simulink model "Bebop10_from_exp"  (R2018a)
settings: Solver=VariableStepAuto  StartTime=0.0  StopTime=100  FixedStep=0.0025  MaxStep=1  MinStep=0.005  RelTol=10  AbsTol=10
values from neighbouring files (symbols this model uses):
  flightplan = [dist,0,height,deg2rad(090) ... (first row only)    [compare_cubic_spline_1.m]    (also in initialize_race_realtime.m = flightplan - [0.5*min(flightplan(:,1:2))+0.5*max(flightplan(; initialize_race_realtime_backup_cubic.m; plot_sim.m = [ 4.348, -0.278, height, deg2rad(  0); test_b_spline.m)
  FOV = 1.05    [initialize_race_realtime_backup_cubic.m]
  g = 9.81    [initialize_race_no_realtime.m]    (also in initialize_race_realtime.m; initialize_race_realtime_backup_cubic.m; moving_average_rls_own.m = P(i-1)*meas*(lambda+meas*P(i-1)*meas)^-1)
  gate_size = 1.4    [initialize_race_realtime.m]    (also in initialize_race_realtime_backup_cubic.m)
  gates = sim_gates(:,:,1)    [eval_sim.m]    (also in initialize_race_realtime.m = flightplan + pert; initialize_race_realtime_backup_cubic.m = [dist,0,height,deg2rad(110); plot_sim.m)
  HFOV = VFOV*resolution(1)/resolution(2)    [initialize_race_realtime.m]
  I = [1 0 0 ... (first row only)    [Bebop_sim_init.m]    (also in initialize_race_no_realtime.m; initialize_race_realtime.m; initialize_race_realtime_backup_cubic.m; moving_averge_rls_download.m = ones(1,N))
  m = 0.68    [calc_plot_spline.m]    (also in calc_spline.m; compare_cubic_spline_1.m = vpasolve(e,r); compare_cubic_spline_2.m = r/3*(-sin(dp)+sqrt(sin(dp)^2-6*cos(dp)+6)); initialize_race_no_realtime.m = 2)
  mass = 2    [Bebop_sim_init.m]    (also in initialize_race_realtime.m = 0.5)
  max_rot_Z = (90)*pi/180    (= 1.57079632679)    [Bebop_sim_init.m]    (also in initialize_race_no_realtime.m = 1.0471975512; initialize_race_realtime.m = 3.14159265359; initialize_race_realtime_backup_cubic.m; run_batch1.m = list_agility(idx_agility)*max_rot_Z)
  max_theta_X = (40)*pi/180    (= 0.698131700798)    [Bebop_sim_init.m]    (also in initialize_race_no_realtime.m = 0.13962634016; initialize_race_realtime.m = 0.418879020479; initialize_race_realtime_backup_cubic.m = 1.308996939; run_batch1.m = list_agility(idx_agility)*max_theta_X)
  max_theta_Y = (40)*pi/180    (= 0.698131700798)    [Bebop_sim_init.m]    (also in initialize_race_no_realtime.m = 0.13962634016; initialize_race_realtime.m = 0.418879020479; initialize_race_realtime_backup_cubic.m = 1.308996939; run_batch1.m = list_agility(idx_agility)*max_theta_Y)
  max_v_Z = .5    (= 0.5)    [Bebop_sim_init.m]    (also in initialize_race_no_realtime.m = 1; initialize_race_realtime.m = 6; initialize_race_realtime_backup_cubic.m = 3; run_batch1.m = list_agility(idx_agility)*max_v_Z)
  max_vel = 2.0    (= 2)    [initialize_race_realtime.m]    (also in initialize_race_realtime_backup_cubic.m = 1.5; run_batch1.m = list_speed(idx_speed); run_batch2.m = list_speed(idx_speed); run_batch3.m = list_speed(idx_speed))
  resolution = 0.5*[1280 720]    [initialize_race_realtime.m]
  spline_init = [P0;P1;P2;P3]    [initialize_race_realtime.m]
  std_dev_eul = 0.25*deg2rad(0.8)*ones(1,3)    [initialize_race_realtime.m]    (also in run_batch1.m = list_sensor_eul(idx_sensor)*dist*ones(1,3); run_batch2.m = list_sensor_eul(idx_sensor)*dist*ones(1,3); run_batch3.m = list_sensor_eul(idx_sensor)*dist*ones(1,3); run_batch4.m = list_sensor_eul(idx_sensor)*dist*ones(1,3))
  std_dev_F = 0.1*max_force*ones(1,3)    [initialize_race_realtime.m]    (also in run_batch1.m = list_actuator(idx_actuator)*max_force*ones(1,3); run_batch2.m = list_actuator(idx_actuator)*max_force*ones(1,3); run_batch3.m = list_actuator(idx_sensor)*max_force*ones(1,3); run_batch4.m = list_actuator(idx_sensor)*max_force*ones(1,3))
  std_dev_M = 0.1*max_moment*[0, 0, 1]    [initialize_race_realtime.m]    (also in run_batch1.m = list_actuator(idx_actuator)*max_moment*[0, 0, 1]; run_batch2.m = list_actuator(idx_actuator)*max_moment*[0, 0, 1]; run_batch3.m = list_actuator(idx_sensor)*max_moment*[0, 0, 1]; run_batch4.m = list_actuator(idx_sensor)*max_moment*[0, 0, 1])
  std_dev_vel = 0.06*ones(1,3)    [initialize_race_realtime.m]    (also in run_batch1.m = list_sensor(idx_sensor)*dist*ones(1,3); run_batch2.m = list_sensor(idx_sensor)*dist*ones(1,3); run_batch3.m = list_sensor(idx_sensor)*dist*ones(1,3); run_batch4.m = list_sensor(idx_sensor)*dist*ones(1,3))
  std_dev_xyz = 0.06*ones(1,3)    [initialize_race_realtime.m]    (also in run_batch1.m = list_sensor(idx_sensor)*dist*ones(1,3); run_batch2.m = list_sensor(idx_sensor)*dist*ones(1,3); run_batch3.m = list_sensor(idx_sensor)*dist*ones(1,3); run_batch4.m = list_sensor(idx_sensor)*dist*ones(1,3))
  two_std_dev_init = [1,1,0.5,deg2rad(30)]    [initialize_race_realtime.m]
  two_std_dev_thres = 0.3    [initialize_race_realtime.m]
  VFOV = 1.05    [initialize_race_realtime.m]
undefined symbols (not defined in the file or in its folder): gray, Rec, SDTV
libraries: sharedtransform x13, visiontextngfix x5, aerolibactuator x4, simulink x3, aerolibutil x2, visionconversions x2, shared6dof x1, vrlib x1, visionanalysis x1, visionstatistics x1, visiontransforms x1
(part 2 of 3)

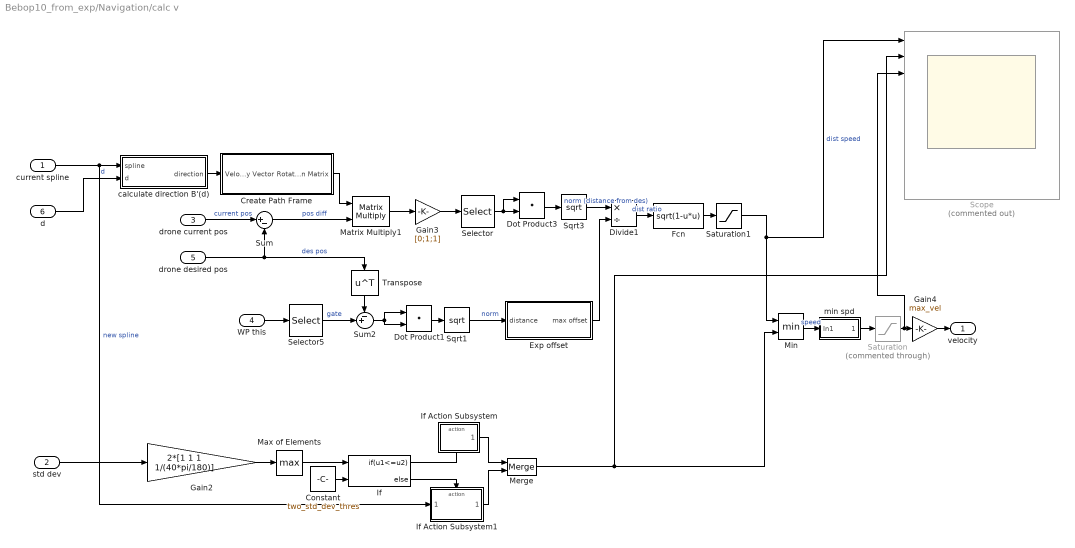
== system Bebop10_from_exp/Navigation/calc v ==
  current spline : Inport
  std dev : Inport  Port=2
  drone current pos : Inport  Port=3
  WP this : Inport  Port=4
  drone desired pos : Inport  Port=5
  d : Inport  Port=6
  Constant : Constant  Value=two_std_dev_thres
  Create Path Frame : Subsystem
  Divide1 : Product  Inputs=*/
  Dot Product1 : DotProduct  InputSameDT=on  OutDataTypeStr=Inherit: Inherit via internal rule
  Dot Product3 : DotProduct  InputSameDT=on  OutDataTypeStr=Inherit: Inherit via internal rule
  Exp offset : Subsystem
  Fcn : Fcn  Expr=sqrt(1-u*u)
  Gain2 : Gain  Gain=2*[1 1 1 1/(40*pi/180)]
  Gain3 : Gain  Gain=[0;1;1]
  Gain4 : Gain  Gain=max_vel
  If : If  NumInputs=2  IfExpression=u1<=u2
  If Action Subsystem : Subsystem  TreatAsAtomicUnit=on
  If Action Subsystem1 : Subsystem  TreatAsAtomicUnit=on
  Matrix Multiply1 : Product  Inputs=**  Multiplication=Matrix(*)
  Max of Elements : MinMax  Function=max
  Merge : Merge
  Min : MinMax  Inputs=2
  Saturation : Saturate  Commented=through  UpperLimit=1.01  LowerLimit=0.99
  Saturation1 : Saturate  UpperLimit=1  LowerLimit=0
  Scope : Scope  Commented=on  NumInputPorts=10
  Selector : Selector  IndexMode=Zero-based  InputPortWidth=3  IndexOptions=Index vector (dialog)  Indices=[0 1 2]  OutputSizes=1
  Selector5 : Selector  NumberOfDimensions=2  IndexMode=Zero-based  InputPortWidth=4  IndexOptions=Select all,Index vector (dialog)  Indices=[1 2 3],[0 1 2]  OutputSizes=1,1
  Sqrt1 : Sqrt  SaturateOnIntegerOverflow=on
  Sqrt3 : Sqrt  SaturateOnIntegerOverflow=on
  Sum : Sum  Inputs=|+-
  Sum2 : Sum  Inputs=-+|
  Transpose : Math  Operator=transpose  SaturateOnIntegerOverflow=on
  calculate direction B'(d) : Subsystem
  min spd : Subsystem
  velocity : Outport
  wires:
  If Action Subsystem1/1(red vel) -> Merge/2
  If Action Subsystem/1(1) -> Merge/1
  If/1 -> If Action Subsystem/Action
  std dev/1 -> Gain2/1
  If/2 -> If Action Subsystem1/Action
  Gain2/1 -> Max of Elements/1
  Max of Elements/1 -> If/1
  Create Path Frame/1(Rotation Matrix) -> Matrix Multiply1/1
  Sum2/1 -> Dot Product1/1, Dot Product1/2
  Min/1 -> min spd/1(In1)  "speed"
  Fcn/1 -> Saturation1/1
  Saturation/1 -> Scope/3, Gain4/1
  Dot Product3/1 -> Sqrt3/1
  Selector5/1 -> Sum2/2  "gate"
  calculate direction B'(d)/1(direction) -> Create Path Frame/1(Velocity Vector)
  Divide1/1 -> Fcn/1  "dist ratio"
  Selector/1 -> Dot Product3/1, Dot Product3/2
  d/1 -> calculate direction B'(d)/2(d)  "d"
  Sum/1 -> Matrix Multiply1/2  "pos diff"
  Merge/1 -> Scope/2, Min/2
  Sqrt1/1 -> Exp offset/1(distance)  "norm"
  Dot Product1/1 -> Sqrt1/1
  drone desired pos/1 -> Transpose/1, Sum/2  "des pos"
  Saturation1/1 -> Scope/1, Min/1  "dist speed"
  Exp offset/1(max offset) -> Divide1/2
  Gain4/1 -> velocity/1
  Sqrt3/1 -> Divide1/1  "norm (distance from des)"
  drone current pos/1 -> Sum/1  "current pos"
  Transpose/1 -> Sum2/1
  min spd/1(Out1) -> Saturation/1
  Matrix Multiply1/1 -> Gain3/1
  current spline/1 -> If Action Subsystem1/1(spline), calculate direction B'(d)/1(spline)  "new spline"
  WP this/1 -> Selector5/1
  Constant/1 -> If/2
  Gain3/1 -> Selector/1

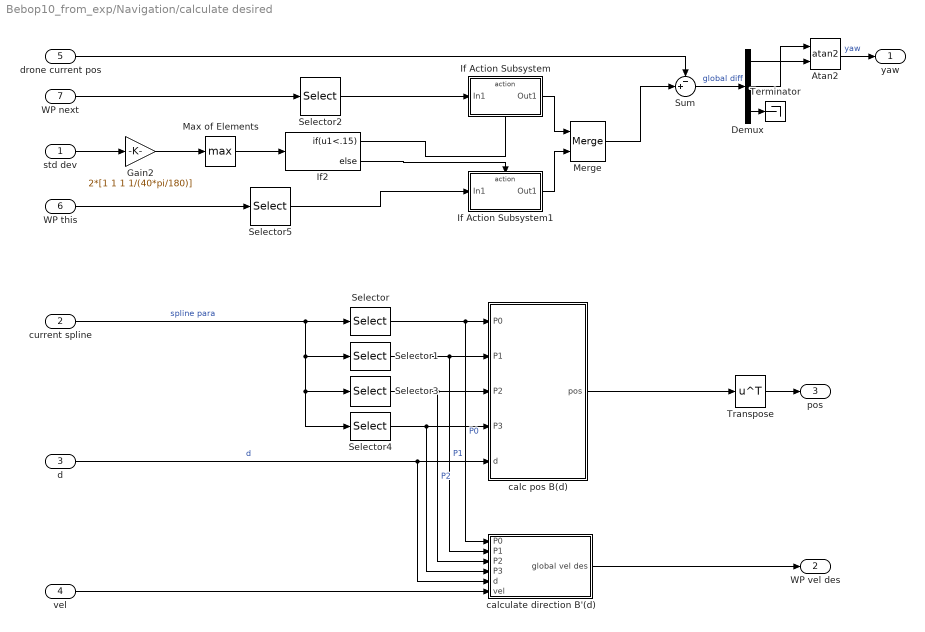
== system Bebop10_from_exp/Navigation/calculate desired ==
  std dev : Inport
  current spline : Inport  Port=2
  d : Inport  Port=3
  vel : Inport  Port=4
  drone current pos : Inport  Port=5
  WP this : Inport  Port=6
  WP next : Inport  Port=7
  Atan2 : Trigonometry  Operator=atan2
  Demux : Demux  Outputs=3
  Gain2 : Gain  Gain=2*[1 1 1 1/(40*pi/180)]
  If Action Subsystem : Subsystem  TreatAsAtomicUnit=on
  If Action Subsystem1 : Subsystem  TreatAsAtomicUnit=on
  If2 : If  IfExpression=u1<.15
  Max of Elements : MinMax  Function=max
  Merge : Merge
  Selector : Selector  NumberOfDimensions=2  IndexMode=Zero-based  InputPortWidth=3  IndexOptions=Index vector (dialog),Select all  Indices=0,[0 1 2]  OutputSizes=1,1
  Selector1 : Selector  NumberOfDimensions=2  IndexMode=Zero-based  InputPortWidth=3  IndexOptions=Index vector (dialog),Select all  Indices=1,[0 1 2]  OutputSizes=1,1
  Selector2 : Selector  NumberOfDimensions=2  IndexMode=Zero-based  InputPortWidth=4  IndexOptions=Select all,Index vector (dialog)  Indices=[1 2 3],[0 1 2]  OutputSizes=1,1
  Selector3 : Selector  NumberOfDimensions=2  IndexMode=Zero-based  InputPortWidth=3  IndexOptions=Index vector (dialog),Select all  Indices=2,[0 1 2]  OutputSizes=1,1
  Selector4 : Selector  NumberOfDimensions=2  IndexMode=Zero-based  InputPortWidth=3  IndexOptions=Index vector (dialog),Select all  Indices=3,[0 1 2]  OutputSizes=1,1
  Selector5 : Selector  NumberOfDimensions=2  IndexMode=Zero-based  InputPortWidth=4  IndexOptions=Select all,Index vector (dialog)  Indices=[1 2 3],[0 1 2]  OutputSizes=1,1
  Sum : Sum  Inputs=-+|
  Terminator : Terminator
  Transpose : Math  Operator=transpose  SaturateOnIntegerOverflow=on
  calc pos B(d) : Subsystem
  calculate direction B'(d) : Subsystem
  yaw : Outport
  WP vel des : Outport  Port=2
  pos : Outport  Port=3
  wires:
  current spline/1 -> Selector4/1, Selector3/1, Selector1/1, Selector/1  "spline para"
  Selector/1 -> calculate direction B'(d)/1(P0), calc pos B(d)/1(P0)  "P0"
  Selector1/1 -> calculate direction B'(d)/2(P1), calc pos B(d)/2(P1)  "P1"
  Selector3/1 -> calculate direction B'(d)/3(P2), calc pos B(d)/3(P2)  "P2"
  d/1 -> calc pos B(d)/5(d), calculate direction B'(d)/5(d)  "d"
  calc pos B(d)/1(pos) -> Transpose/1
  Sum/1 -> Demux/1  "global diff"
  Demux/2 -> Atan2/1
  Demux/1 -> Atan2/2
  Demux/3 -> Terminator/1
  Atan2/1 -> yaw/1  "yaw"
  vel/1 -> calculate direction B'(d)/6(vel)
  calculate direction B'(d)/1(global vel des) -> WP vel des/1
  Transpose/1 -> pos/1
  drone current pos/1 -> Sum/1
  WP next/1 -> Selector2/1
  If Action Subsystem/1(Out1) -> Merge/1
  If Action Subsystem1/1(Out1) -> Merge/2
  WP this/1 -> Selector5/1
  Selector2/1 -> If Action Subsystem/1(In1)
  Selector4/1 -> calc pos B(d)/4(P3), calculate direction B'(d)/4(P3)
  Merge/1 -> Sum/2
  std dev/1 -> Gain2/1
  Gain2/1 -> Max of Elements/1
  Max of Elements/1 -> If2/1
  If2/1 -> If Action Subsystem/Action
  Selector5/1 -> If Action Subsystem1/1(In1)
  If2/2 -> If Action Subsystem1/Action

== system Bebop10_from_exp/Navigation/get WPts ==
  list : Inport
  idx : Inport  Port=2
  Fcn : Fcn  Expr=u-1
  Fcn1 : Fcn  Expr=u+1
  Mod : Math  Operator=mod  SaturateOnIntegerOverflow=on
  Mod1 : Math  Operator=mod  SaturateOnIntegerOverflow=on
  Mod2 : Math  Operator=mod  SaturateOnIntegerOverflow=on
  Probe Dimension : Probe  ProbeWidth=off  ProbeSampleTime=off  ProbeComplexSignal=off  ProbeSignalDimensions=on
  Selector : Selector  InputPortWidth=2  IndexOptions=Index vector (dialog)  Indices=1  OutputSizes=1
  Selector1 : Selector  NumberOfDimensions=2  IndexMode=Zero-based  InputPortWidth=3  IndexOptions=Index vector (port),Select all  Indices=[1 3],1  OutputSizes=1,1
  Selector2 : Selector  NumberOfDimensions=2  IndexMode=Zero-based  InputPortWidth=3  IndexOptions=Index vector (port),Select all  Indices=[1 3],1  OutputSizes=1,1
  Selector3 : Selector  NumberOfDimensions=2  IndexMode=Zero-based  InputPortWidth=3  IndexOptions=Index vector (port),Select all  Indices=[1 3],1  OutputSizes=1,1
  WP last : Outport
  WP this : Outport  Port=2
  WP next : Outport  Port=3
  wires:
  list/1 -> Selector3/1, Selector2/1, Selector1/1, Probe Dimension/1
  idx/1 -> Fcn/1, Mod1/1, Fcn1/1
  Fcn/1 -> Mod/1
  Mod/1 -> Selector1/2
  Fcn1/1 -> Mod2/1
  Probe Dimension/1 -> Selector/1
  Selector/1 -> Mod2/2, Mod1/2, Mod/2
  Mod1/1 -> Selector2/2
  Mod2/1 -> Selector3/2
  Selector1/1 -> WP last/1
  Selector2/1 -> WP this/1
  Selector3/1 -> WP next/1

== system Bebop10_from_exp/Navigation/set position ==
  current spline : Inport
  velocity : Inport  Port=2
  d old : Inport  Port=3
  auto : Inport  Port=4
  Constant2 : Constant
  Mod1 : Math  Operator=mod  SaturateOnIntegerOverflow=on
  Selector10 : Selector  NumberOfDimensions=2  IndexMode=Zero-based  InputPortWidth=3  IndexOptions=Index vector (dialog),Select all  Indices=1,[0 1 2]  OutputSizes=1,1
  Selector11 : Selector  NumberOfDimensions=2  IndexMode=Zero-based  InputPortWidth=3  IndexOptions=Index vector (dialog),Select all  Indices=2,[0 1 2]  OutputSizes=1,1
  Selector12 : Selector  NumberOfDimensions=2  IndexMode=Zero-based  InputPortWidth=3  IndexOptions=Index vector (dialog),Select all  Indices=3,[0 1 2]  OutputSizes=1,1
  Selector7 : Selector  NumberOfDimensions=2  IndexMode=Zero-based  InputPortWidth=3  IndexOptions=Index vector (dialog),Select all  Indices=0,[0 1 2]  OutputSizes=1,1
  Unit Delay2 : UnitDelay  SampleTime=-1
  new d with linearization : Subsystem
  d old1 : Outport
  d new raw : Outport  Port=2
  wires:
  current spline/1 -> Selector7/1, Selector10/1, Selector11/1, Selector12/1  "spline para"
  Selector7/1 -> new d with linearization/3(P0)  "P0"
  Selector10/1 -> new d with linearization/4(P1)  "P1"
  Selector11/1 -> new d with linearization/5(P2)  "P2"
  Selector12/1 -> new d with linearization/6(P3)  "P3"
  d old/1 -> new d with linearization/2(d old)
  velocity/1 -> new d with linearization/1(vel)
  new d with linearization/1(d new same spline) -> d new raw/1, Mod1/1  "d new over"
  Mod1/1 -> Unit Delay2/1
  Constant2/1 -> Mod1/2
  Unit Delay2/1 -> d old1/1
  auto/1 -> new d with linearization/7(auto)

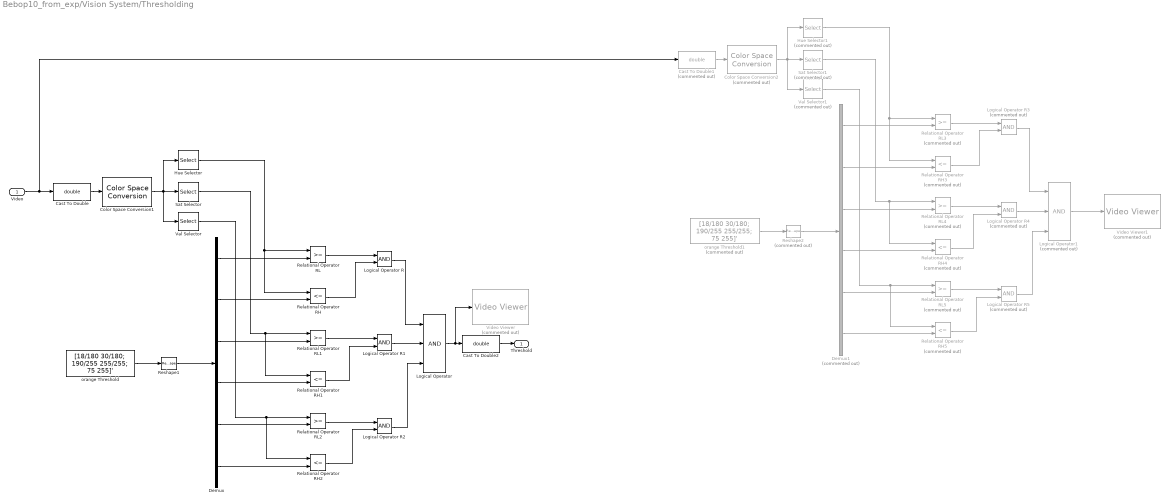
== system Bebop10_from_exp/Vision System/Thresholding ==
  "Video " : Inport
  Cast To Double : DataTypeConversion  OutDataTypeStr=double
  Cast To Double1 : DataTypeConversion  Commented=on  OutDataTypeStr=double
  Cast To Double2 : DataTypeConversion  OutDataTypeStr=double
  Color Space Conversion1 : visionconversions/Color Space  Conversion  conversion=Obsolete  conversionActive=R'G'B' to HSV  wp_str=D65  rec=Rec. 601 (SDTV)  sys=1125/60/2:1  imagePorts=One multidimensional signal
      settings: SourceProductName=Computer Vision System Toolbox
  Color Space Conversion2 : visionconversions/Color Space  Conversion  Commented=on  conversion=Obsolete  conversionActive=R'G'B' to HSV  wp_str=D65  rec=Rec. 601 (SDTV)  sys=1125/60/2:1  imagePorts=One multidimensional signal
      settings: SourceProductName=Computer Vision System Toolbox
  Demux : Demux  Outputs=6
  Demux1 : Demux  Commented=on  Outputs=6
  Hue Selector : Selector  NumberOfDimensions=3  IndexMode=Zero-based  InputPortWidth=3  IndexOptions=Select all,Select all,Index vector (dialog)  Indices=[1 3],1,0  OutputSizes=1,1,1
  Hue Selector1 : Selector  Commented=on  NumberOfDimensions=3  InputPortWidth=3  IndexOptions=Select all,Select all,Index vector (dialog)  Indices=[1 3],1,1  OutputSizes=1,1,1
  Logical Operator : Logic  Inputs=3  AllPortsSameDT=off  OutDataTypeStr=boolean
  Logical Operator R : Logic  AllPortsSameDT=off  OutDataTypeStr=boolean
  Logical Operator R1 : Logic  AllPortsSameDT=off  OutDataTypeStr=boolean
  Logical Operator R2 : Logic  AllPortsSameDT=off  OutDataTypeStr=boolean
  Logical Operator R3 : Logic  Commented=on  AllPortsSameDT=off  OutDataTypeStr=boolean
  Logical Operator R4 : Logic  Commented=on  AllPortsSameDT=off  OutDataTypeStr=boolean
  Logical Operator R5 : Logic  Commented=on  AllPortsSameDT=off  OutDataTypeStr=boolean
  Logical Operator1 : Logic  Commented=on  Inputs=3  AllPortsSameDT=off  OutDataTypeStr=boolean
  Relational Operator RH : RelationalOperator  Operator=<=  OutDataTypeStr=boolean  RndMeth=Nearest
  Relational Operator RH1 : RelationalOperator  Operator=<=  OutDataTypeStr=boolean  RndMeth=Nearest
  Relational Operator RH2 : RelationalOperator  Operator=<=  OutDataTypeStr=boolean  RndMeth=Nearest
  Relational Operator RH3 : RelationalOperator  Commented=on  Operator=<=  OutDataTypeStr=boolean  RndMeth=Nearest
  Relational Operator RH4 : RelationalOperator  Commented=on  Operator=<=  OutDataTypeStr=boolean  RndMeth=Nearest
  Relational Operator RH5 : RelationalOperator  Commented=on  Operator=<=  OutDataTypeStr=boolean  RndMeth=Nearest
  Relational Operator RL : RelationalOperator  OutDataTypeStr=boolean  RndMeth=Nearest
  Relational Operator RL1 : RelationalOperator  OutDataTypeStr=boolean  RndMeth=Nearest
  Relational Operator RL2 : RelationalOperator  OutDataTypeStr=boolean  RndMeth=Nearest
  Relational Operator RL3 : RelationalOperator  Commented=on  OutDataTypeStr=boolean  RndMeth=Nearest
  Relational Operator RL4 : RelationalOperator  Commented=on  OutDataTypeStr=boolean  RndMeth=Nearest
  Relational Operator RL5 : RelationalOperator  Commented=on  OutDataTypeStr=boolean  RndMeth=Nearest
  Reshape1 : Reshape
  Reshape2 : Reshape  Commented=on
  Sat Selector : Selector  NumberOfDimensions=3  IndexMode=Zero-based  InputPortWidth=3  IndexOptions=Select all,Select all,Index vector (dialog)  Indices=[1 3],1,1  OutputSizes=1,1,1
  Sat Selector1 : Selector  Commented=on  NumberOfDimensions=3  InputPortWidth=3  IndexOptions=Select all,Select all,Index vector (dialog)  Indices=[1 3],1,2  OutputSizes=1,1,1
  Val Selector : Selector  NumberOfDimensions=3  IndexMode=Zero-based  InputPortWidth=3  IndexOptions=Select all,Select all,Index vector (dialog)  Indices=[1 3],1,2  OutputSizes=1,1,1
  Val Selector1 : Selector  Commented=on  NumberOfDimensions=3  InputPortWidth=3  IndexOptions=Select all,Select all,Index vector (dialog)  Indices=[1 3],1,3  OutputSizes=1,1,1
  Video Viewer : VideoViewer  Commented=on  colormapValue=gray(256)  FigPos=[833 898 768 793]
  Video Viewer1 : VideoViewer  Commented=on  colormapValue=gray(256)  FigPos=[823 898 778 793]
  orange Threshold : Constant  Value=[18/180 30/180; 190/255 255/255; 75 255]'  OutDataTypeStr=double
  orange Threshold1 : Constant  Commented=on  Value=[18/180 30/180; 190/255 255/255; 75 255]'  OutDataTypeStr=double
  Threshold : Outport
  wires:
  Color Space Conversion1/1 -> Val Selector/1, Sat Selector/1, Hue Selector/1
  Demux/6 -> Relational Operator RH2/2
  Val Selector/1 -> Relational Operator RH2/1, Relational Operator RL2/1
  Demux/3 -> Relational Operator RL1/2
  Relational Operator RL/1 -> Logical Operator R/1
  Demux/2 -> Relational Operator RH/2
  orange Threshold/1 -> Reshape1/1
  Cast To Double/1 -> Color Space Conversion1/1
  Demux/5 -> Relational Operator RL2/2
  Hue Selector/1 -> Relational Operator RH/1, Relational Operator RL/1
  Logical Operator R/1 -> Logical Operator/1
  Relational Operator RH/1 -> Logical Operator R/2
  Demux/1 -> Relational Operator RL/2
  Demux/4 -> Relational Operator RH1/2
  Reshape1/1 -> Demux/1
  Logical Operator R1/1 -> Logical Operator/2
  Relational Operator RH1/1 -> Logical Operator R1/2
  Sat Selector/1 -> Relational Operator RH1/1, Relational Operator RL1/1
  Relational Operator RL1/1 -> Logical Operator R1/1
  Relational Operator RH2/1 -> Logical Operator R2/2
  Relational Operator RL2/1 -> Logical Operator R2/1
  Logical Operator R2/1 -> Logical Operator/3
  Logical Operator/1 -> Video Viewer/1, Cast To Double2/1
  Demux1/5 -> Relational Operator RL5/2
  Relational Operator RH3/1 -> Logical Operator R3/2
  orange Threshold1/1 -> Reshape2/1
  Demux1/1 -> Relational Operator RL3/2
  Relational Operator RH4/1 -> Logical Operator R4/2
  Demux1/4 -> Relational Operator RH4/2
  Relational Operator RH5/1 -> Logical Operator R5/2
  Logical Operator R5/1 -> Logical Operator1/3
  Relational Operator RL4/1 -> Logical Operator R4/1
  Demux1/6 -> Relational Operator RH5/2
  Demux1/2 -> Relational Operator RH3/2
  Reshape2/1 -> Demux1/1
  Logical Operator1/1 -> Video Viewer1/1
  Hue Selector1/1 -> Relational Operator RH3/1, Relational Operator RL3/1
  Color Space Conversion2/1 -> Val Selector1/1, Sat Selector1/1, Hue Selector1/1
  Logical Operator R3/1 -> Logical Operator1/1
  Cast To Double1/1 -> Color Space Conversion2/1
  Demux1/3 -> Relational Operator RL4/2
  Relational Operator RL3/1 -> Logical Operator R3/1
  Val Selector1/1 -> Relational Operator RH5/1, Relational Operator RL5/1
  Relational Operator RL5/1 -> Logical Operator R5/1
  Logical Operator R4/1 -> Logical Operator1/2
  "Video "/1 -> Cast To Double1/1, Cast To Double/1
  Sat Selector1/1 -> Relational Operator RH4/1, Relational Operator RL4/1
  Cast To Double2/1 -> Threshold/1

== system Bebop10_from_exp/Vision System/show all lines ==
  original image : Inport
  lines : Inport  Port=2
  pts : Inport  Port=3
  Cast To Double : DataTypeConversion  OutDataTypeStr=int32
  Cast To Double1 : DataTypeConversion  OutDataTypeStr=int32
  Draw Markers2 : visiontextngfix/Draw Markers  shape=Circle  size=3  fill=on  fillClrSource=Specify via dialog  display=Black  intensity=200  color=[200 255 100]  opacity=1  viewport=Entire image  antialiasing=off  inType=Obsolete  imagePorts=One multidimensional signal  prodOutputMode=Binary point scaling  prodOutputWordLength=32  prodOutputFracLength=14  memoryMode=Specify word length  memoryWordLength=16  memoryFracLength=14  roundingMode=Floor  overflowMode=off
      settings: SourceProductName=Computer Vision System Toolbox  SourceProductBaseCode=VP
  Draw Shapes : visiontextngfix/Draw Shapes  shape=Lines  fill=off  lineWidth=1  fillClrSource=Specify via dialog  display=White  intensity=200  color=[200 255 100]  opacity=0.6  viewport=Entire image  antialiasing=off  inType=Obsolete  imagePorts=One multidimensional signal  prodOutputMode=Binary point scaling  prodOutputWordLength=32  prodOutputFracLength=14  memoryMode=Specify word length  memoryWordLength=16  memoryFracLength=14  roundingMode=Floor  overflowMode=off
      settings: SourceProductName=Computer Vision System Toolbox
  Video Viewer3 : VideoViewer  colormapValue=gray(256)  FigPos=[66 1078 1855 973]
  wires:
  original image/1 -> Draw Shapes/1
  Draw Shapes/1 -> Draw Markers2/1
  lines/1 -> Cast To Double/1
  pts/1 -> Cast To Double1/1
  Cast To Double/1 -> Draw Shapes/2
  Draw Markers2/1 -> Video Viewer3/1
  Cast To Double1/1 -> Draw Markers2/2

== system Bebop10_from_exp/Vision System/show feature lines ==
  original image : Inport
  lines : Inport  Port=2
  pts : Inport  Port=3
  Cast To Double : DataTypeConversion  OutDataTypeStr=int32
  Cast To Double1 : DataTypeConversion  OutDataTypeStr=int32
  Draw Markers2 : visiontextngfix/Draw Markers  shape=Circle  size=3  fill=on  fillClrSource=Specify via dialog  display=Black  intensity=200  color=[200 255 100]  opacity=1  viewport=Entire image  antialiasing=off  inType=Obsolete  imagePorts=One multidimensional signal  prodOutputMode=Binary point scaling  prodOutputWordLength=32  prodOutputFracLength=14  memoryMode=Specify word length  memoryWordLength=16  memoryFracLength=14  roundingMode=Floor  overflowMode=off
      settings: SourceProductName=Computer Vision System Toolbox  SourceProductBaseCode=VP
  Draw Shapes : visiontextngfix/Draw Shapes  shape=Lines  fill=off  lineWidth=1  fillClrSource=Specify via dialog  display=White  intensity=200  color=[200 255 100]  opacity=0.6  viewport=Entire image  antialiasing=off  inType=Obsolete  imagePorts=One multidimensional signal  prodOutputMode=Binary point scaling  prodOutputWordLength=32  prodOutputFracLength=14  memoryMode=Specify word length  memoryWordLength=16  memoryFracLength=14  roundingMode=Floor  overflowMode=off
      settings: SourceProductName=Computer Vision System Toolbox
  Video Viewer3 : VideoViewer  colormapValue=gray(256)  FigPos=[66 1078 928 945]
  wires:
  original image/1 -> Draw Shapes/1
  Draw Shapes/1 -> Draw Markers2/1
  lines/1 -> Cast To Double/1
  pts/1 -> Cast To Double1/1
  Cast To Double/1 -> Draw Shapes/2
  Draw Markers2/1 -> Video Viewer3/1
  Cast To Double1/1 -> Draw Markers2/2

== system Bebop10_from_exp/Vision System/show gate ==
  original image : Inport
  gate pts : Inport  Port=2
  Draw Markers1 : visiontextngfix/Draw Markers  shape=Circle  size=10  fill=on  fillClrSource=Specify via dialog  display=White  intensity=200  color=[200 255 100]  opacity=1  viewport=Entire image  antialiasing=off  inType=Obsolete  imagePorts=One multidimensional signal  prodOutputMode=Binary point scaling  prodOutputWordLength=32  prodOutputFracLength=14  memoryMode=Specify word length  memoryWordLength=16  memoryFracLength=14  roundingMode=Floor  overflowMode=off
      settings: SourceProductName=Computer Vision System Toolbox  SourceProductBaseCode=VP
  Video Viewer1 : VideoViewer  colormapValue=gray(256)  FigPos=[1104 1072 735 551]
  wires:
  gate pts/1 -> Draw Markers1/2
  Draw Markers1/1 -> Video Viewer1/1
  original image/1 -> Draw Markers1/1

== system Bebop10_from_exp/conv/global2strange drone ==
  note: rotm2axang(m1*m2)
  note: eul2rotm([-pi/2, 0, pi/2])
  note: eul2rotm([euler(3),euler(2),euler(1)])
  euler global : Inport
  Constant : Constant  Value=pi/2
  Constant1 : Constant  Value=0
  Direction Cosine Matrix to Quaternions : sharedtransform/Direction Cosine Matrix  to Quaternions  aMode=0  action=None  tolerance=eps(2)
      settings: SourceProductName=Aerospace Blockset  SourceProductBaseCode=AE
  Gain : Gain  Gain=-1
  Gain2 : Gain  Gain=-1
  Gain3 : Gain  Gain=[-1,-1,-1,1]
  MATLAB Function : MATLAB Function  Commented=on  TreatAsAtomicUnit=on
  MATLAB Function1 : MATLAB Function  TreatAsAtomicUnit=on
  Matrix Multiply : Product  Multiplication=Matrix(*)
  Rotation Angles to Direction Cosine Matrix : sharedtransform/Rotation Angles to Direction Cosine Matrix  rotationOrder=XYZ  aMode=aMode
      settings: SourceProductBaseCode=AE
  Rotation Angles to Direction Cosine Matrix1 : sharedtransform/Rotation Angles to Direction Cosine Matrix  rotationOrder=XYZ  aMode=aMode
      settings: SourceProductBaseCode=AE
  Vector Concatenate : Concatenate  NumInputs=3
  axang strange : Outport
  wires:
  Constant/1 -> Vector Concatenate/3, Gain/1
  Constant1/1 -> Vector Concatenate/2
  Gain/1 -> Vector Concatenate/1
  Rotation Angles to Direction Cosine Matrix/1 -> Matrix Multiply/2
  euler global/1 -> Gain2/1
  Rotation Angles to Direction Cosine Matrix1/1 -> Matrix Multiply/1
  Matrix Multiply/1 -> Direction Cosine Matrix to Quaternions/1
  MATLAB Function1/1(axang) -> Gain3/1
  Vector Concatenate/1 -> Rotation Angles to Direction Cosine Matrix/1
  Gain2/1 -> Rotation Angles to Direction Cosine Matrix1/1
  Direction Cosine Matrix to Quaternions/1 -> MATLAB Function1/1(q)
  Gain3/1 -> axang strange/1

== system Bebop10_from_exp/Control/Create Path Frame/Make X Vector ==
  Velocity Vector : Inport
  Make Unit : Subsystem
  X Vector : Outport
  wires:
  Velocity Vector/1 -> Make Unit/1(Vector)
  Make Unit/1(Unit Vector) -> X Vector/1

== system Bebop10_from_exp/Control/Create Path Frame/Make Y Vector ==
  Velocity Vector : Inport
  Constant : Constant  Value=0
  Demux : Demux  Outputs=3
  Gain : Gain  Gain=-1
  Make Unit : Subsystem
  Matrix Concatenate : Concatenate  NumInputs=3  Mode=Multidimensional array
  Terminator : Terminator
  Y Vector : Outport
  wires:
  Make Unit/1(Unit Vector) -> Y Vector/1
  Velocity Vector/1 -> Demux/1
  Demux/3 -> Terminator/1
  Demux/2 -> Gain/1
  Gain/1 -> Matrix Concatenate/1
  Demux/1 -> Matrix Concatenate/2
  Constant/1 -> Matrix Concatenate/3
  Matrix Concatenate/1 -> Make Unit/1(Vector)

== system Bebop10_from_exp/Control/Create Path Frame/Make Z Vector ==
  Velocity Vector : Inport
  Add : Sum
  Demux : Demux  Outputs=3
  Gain : Gain  Gain=-1
  Gain1 : Gain  Gain=-1
  Make Unit : Subsystem
  Matrix Concatenate : Concatenate  NumInputs=3  Mode=Multidimensional array
  Multiply : Product
  Multiply1 : Product
  Square : Math  Operator=square  SaturateOnIntegerOverflow=on
  Square1 : Math  Operator=square  SaturateOnIntegerOverflow=on
  Z Vector : Outport
  wires:
  Make Unit/1(Unit Vector) -> Z Vector/1
  Velocity Vector/1 -> Demux/1
  Demux/3 -> Multiply/2, Multiply1/2
  Matrix Concatenate/1 -> Make Unit/1(Vector)
  Multiply/1 -> Gain/1
  Gain/1 -> Matrix Concatenate/1
  Demux/1 -> Square/1, Multiply/1
  Multiply1/1 -> Gain1/1
  Gain1/1 -> Matrix Concatenate/2
  Demux/2 -> Square1/1, Multiply1/1
  Add/1 -> Matrix Concatenate/3
  Square/1 -> Add/1
  Square1/1 -> Add/2

== system Bebop10_from_exp/Control/Subsystem/ctrl r ==
  P : Inport
  D : Inport  Port=2
  Value : Inport  Port=3
  Add : Sum  Inputs=+++
  Add1 : Sum
  Gain : Gain  Gain=3
  Gain1 : Gain
  Gain2 : Gain  Gain=2
  Gain3 : Gain  Gain=0.1
  Multiply : Product
  Multiply1 : Product
  Sum : Sum  Inputs=-+|
  Sum1 : Sum  Inputs=-+|
  Sum2 : Sum  Inputs=-+|
  Unit Delay1 : UnitDelay  SampleTime=-1
  Unit Delay2 : UnitDelay  SampleTime=-1
  Unit Delay3 : UnitDelay  SampleTime=-1
  Acc : Outport
  wires:
  Unit Delay1/1 -> Sum/1, Unit Delay2/1
  Multiply1/1 -> Add1/2  "P"
  Multiply/1 -> Sum/2, Sum1/2, Sum2/2, Unit Delay1/1
  Gain3/1 -> Add1/1  "D"
  Unit Delay2/1 -> Sum1/1, Unit Delay3/1
  Value/1 -> Multiply1/1, Multiply/2
  Unit Delay3/1 -> Sum2/1
  Add1/1 -> Acc/1
  D/1 -> Multiply/1
  P/1 -> Multiply1/2
  Sum2/1 -> Gain1/1
  Sum1/1 -> Gain2/1
  Sum/1 -> Gain/1
  Gain1/1 -> Add/1
  Gain2/1 -> Add/2
  Gain/1 -> Add/3
  Add/1 -> Gain3/1

== system Bebop10_from_exp/Control/Subsystem/ctrl x ==
  P : Inport
  D : Inport  Port=2
  Value : Inport  Port=3
  Add : Sum  Inputs=+++
  Add1 : Sum
  Gain : Gain  Gain=3
  Gain1 : Gain
  Gain2 : Gain  Gain=2
  Gain3 : Gain  Gain=0.1
  Multiply : Product
  Multiply1 : Product
  Scope : Scope  NumInputPorts=2
  Sum : Sum  Inputs=-+|
  Sum1 : Sum  Inputs=-+|
  Sum2 : Sum  Inputs=-+|
  Unit Delay1 : UnitDelay  SampleTime=-1
  Unit Delay2 : UnitDelay  SampleTime=-1
  Unit Delay3 : UnitDelay  SampleTime=-1
  Acc : Outport
  wires:
  Unit Delay1/1 -> Sum/1, Unit Delay2/1
  Multiply1/1 -> Scope/2, Add1/2  "P"
  Multiply/1 -> Sum/2, Sum1/2, Sum2/2, Unit Delay1/1
  Gain3/1 -> Scope/1, Add1/1  "D"
  Unit Delay2/1 -> Sum1/1, Unit Delay3/1
  Value/1 -> Multiply1/1, Multiply/2
  Unit Delay3/1 -> Sum2/1
  Add1/1 -> Acc/1
  D/1 -> Multiply/1
  P/1 -> Multiply1/2
  Sum2/1 -> Gain1/1
  Sum1/1 -> Gain2/1
  Sum/1 -> Gain/1
  Gain1/1 -> Add/1
  Gain2/1 -> Add/2
  Gain/1 -> Add/3
  Add/1 -> Gain3/1

== system Bebop10_from_exp/Control/Subsystem/ctrl y ==
  P : Inport
  D : Inport  Port=2
  Value : Inport  Port=3
  Add : Sum  Inputs=+++
  Add1 : Sum
  Gain : Gain  Gain=3
  Gain1 : Gain
  Gain2 : Gain  Gain=2
  Gain3 : Gain  Gain=0.1
  Multiply : Product
  Multiply1 : Product
  Sum : Sum  Inputs=-+|
  Sum1 : Sum  Inputs=-+|
  Sum2 : Sum  Inputs=-+|
  Unit Delay1 : UnitDelay  SampleTime=-1
  Unit Delay2 : UnitDelay  SampleTime=-1
  Unit Delay3 : UnitDelay  SampleTime=-1
  Acc : Outport
  wires:
  Unit Delay1/1 -> Sum/1, Unit Delay2/1
  Multiply1/1 -> Add1/2  "P"
  Multiply/1 -> Sum/2, Sum1/2, Sum2/2, Unit Delay1/1
  Gain3/1 -> Add1/1  "D"
  Unit Delay2/1 -> Sum1/1, Unit Delay3/1
  Value/1 -> Multiply1/1, Multiply/2
  Unit Delay3/1 -> Sum2/1
  Add1/1 -> Acc/1
  D/1 -> Multiply/1
  P/1 -> Multiply1/2
  Sum2/1 -> Gain1/1
  Sum1/1 -> Gain2/1
  Sum/1 -> Gain/1
  Gain1/1 -> Add/1
  Gain2/1 -> Add/2
  Gain/1 -> Add/3
  Add/1 -> Gain3/1

== system Bebop10_from_exp/Control/Subsystem/ctrl z ==
  P : Inport
  D : Inport  Port=2
  Value : Inport  Port=3
  Add : Sum  Inputs=+++
  Add1 : Sum
  Gain : Gain  Gain=3
  Gain1 : Gain
  Gain2 : Gain  Gain=2
  Gain3 : Gain  Gain=0.1
  Multiply : Product
  Multiply1 : Product
  Sum : Sum  Inputs=-+|
  Sum1 : Sum  Inputs=-+|
  Sum2 : Sum  Inputs=-+|
  Unit Delay1 : UnitDelay  SampleTime=-1
  Unit Delay2 : UnitDelay  SampleTime=-1
  Unit Delay3 : UnitDelay  SampleTime=-1
  Acc : Outport
  wires:
  Unit Delay1/1 -> Sum/1, Unit Delay2/1
  Multiply1/1 -> Add1/2  "P"
  Multiply/1 -> Sum/2, Sum1/2, Sum2/2, Unit Delay1/1
  Gain3/1 -> Add1/1  "D"
  Unit Delay2/1 -> Sum1/1, Unit Delay3/1
  Value/1 -> Multiply1/1, Multiply/2
  Unit Delay3/1 -> Sum2/1
  Add1/1 -> Acc/1
  D/1 -> Multiply/1
  P/1 -> Multiply1/2
  Sum2/1 -> Gain1/1
  Sum1/1 -> Gain2/1
  Sum/1 -> Gain/1
  Gain1/1 -> Add/1
  Gain2/1 -> Add/2
  Gain/1 -> Add/3
  Add/1 -> Gain3/1

== system Bebop10_from_exp/Gate info/Yaw2Axang1/Subsystem ==
  note: u(2)/sqrt(1-u(1)*u(1)), u(3)/sqrt(1-u(1)*u(1)), u(4)/sqrt(1-u(1)*u(1)),
  In1 : Inport
  Fcn : Fcn  Expr=2*acos(u(1))
  Fcn1 : Fcn  Expr=u(2)/sqrt(1-u(1)*u(1))
  Fcn2 : Fcn  Expr=u(3)/sqrt(1-u(1)*u(1))
  Fcn3 : Fcn  Expr=u(4)/sqrt(1-u(1)*u(1))
  Vector Concatenate : Concatenate  NumInputs=4
  Out1 : Outport
  wires:
  In1/1 -> Fcn/1, Fcn3/1, Fcn2/1, Fcn1/1
  Fcn1/1 -> Vector Concatenate/1
  Fcn2/1 -> Vector Concatenate/2
  Fcn3/1 -> Vector Concatenate/3
  Fcn/1 -> Vector Concatenate/4
  Vector Concatenate/1 -> Out1/1

== system Bebop10_from_exp/Gate info/Yaw2Axang2/Subsystem ==
  note: u(2)/sqrt(1-u(1)*u(1)), u(3)/sqrt(1-u(1)*u(1)), u(4)/sqrt(1-u(1)*u(1)),
  In1 : Inport
  Fcn : Fcn  Expr=2*acos(u(1))
  Fcn1 : Fcn  Expr=u(2)/sqrt(1-u(1)*u(1))
  Fcn2 : Fcn  Expr=u(3)/sqrt(1-u(1)*u(1))
  Fcn3 : Fcn  Expr=u(4)/sqrt(1-u(1)*u(1))
  Vector Concatenate : Concatenate  NumInputs=4
  Out1 : Outport
  wires:
  In1/1 -> Fcn/1, Fcn3/1, Fcn2/1, Fcn1/1
  Fcn1/1 -> Vector Concatenate/1
  Fcn2/1 -> Vector Concatenate/2
  Fcn3/1 -> Vector Concatenate/3
  Fcn/1 -> Vector Concatenate/4
  Vector Concatenate/1 -> Out1/1

== system Bebop10_from_exp/Gate info/Yaw2Axang3/Subsystem ==
  note: u(2)/sqrt(1-u(1)*u(1)), u(3)/sqrt(1-u(1)*u(1)), u(4)/sqrt(1-u(1)*u(1)),
  In1 : Inport
  Fcn : Fcn  Expr=2*acos(u(1))
  Fcn1 : Fcn  Expr=u(2)/sqrt(1-u(1)*u(1))
  Fcn2 : Fcn  Expr=u(3)/sqrt(1-u(1)*u(1))
  Fcn3 : Fcn  Expr=u(4)/sqrt(1-u(1)*u(1))
  Vector Concatenate : Concatenate  NumInputs=4
  Out1 : Outport
  wires:
  In1/1 -> Fcn/1, Fcn3/1, Fcn2/1, Fcn1/1
  Fcn1/1 -> Vector Concatenate/1
  Fcn2/1 -> Vector Concatenate/2
  Fcn3/1 -> Vector Concatenate/3
  Fcn/1 -> Vector Concatenate/4
  Vector Concatenate/1 -> Out1/1

== system Bebop10_from_exp/Gate info/Yaw2Axang4/Subsystem ==
  note: u(2)/sqrt(1-u(1)*u(1)), u(3)/sqrt(1-u(1)*u(1)), u(4)/sqrt(1-u(1)*u(1)),
  In1 : Inport
  Fcn : Fcn  Expr=2*acos(u(1))
  Fcn1 : Fcn  Expr=u(2)/sqrt(1-u(1)*u(1))
  Fcn2 : Fcn  Expr=u(3)/sqrt(1-u(1)*u(1))
  Fcn3 : Fcn  Expr=u(4)/sqrt(1-u(1)*u(1))
  Vector Concatenate : Concatenate  NumInputs=4
  Out1 : Outport
  wires:
  In1/1 -> Fcn/1, Fcn3/1, Fcn2/1, Fcn1/1
  Fcn1/1 -> Vector Concatenate/1
  Fcn2/1 -> Vector Concatenate/2
  Fcn3/1 -> Vector Concatenate/3
  Fcn/1 -> Vector Concatenate/4
  Vector Concatenate/1 -> Out1/1

== system Bebop10_from_exp/Gate info/Yaw2Axang5/Subsystem ==
  note: u(2)/sqrt(1-u(1)*u(1)), u(3)/sqrt(1-u(1)*u(1)), u(4)/sqrt(1-u(1)*u(1)),
  In1 : Inport
  Fcn : Fcn  Expr=2*acos(u(1))
  Fcn1 : Fcn  Expr=u(2)/sqrt(1-u(1)*u(1))
  Fcn2 : Fcn  Expr=u(3)/sqrt(1-u(1)*u(1))
  Fcn3 : Fcn  Expr=u(4)/sqrt(1-u(1)*u(1))
  Vector Concatenate : Concatenate  NumInputs=4
  Out1 : Outport
  wires:
  In1/1 -> Fcn/1, Fcn3/1, Fcn2/1, Fcn1/1
  Fcn1/1 -> Vector Concatenate/1
  Fcn2/1 -> Vector Concatenate/2
  Fcn3/1 -> Vector Concatenate/3
  Fcn/1 -> Vector Concatenate/4
  Vector Concatenate/1 -> Out1/1

== system Bebop10_from_exp/Gate info/Yaw2Axang6/Subsystem ==
  note: u(2)/sqrt(1-u(1)*u(1)), u(3)/sqrt(1-u(1)*u(1)), u(4)/sqrt(1-u(1)*u(1)),
  In1 : Inport
  Fcn : Fcn  Expr=2*acos(u(1))
  Fcn1 : Fcn  Expr=u(2)/sqrt(1-u(1)*u(1))
  Fcn2 : Fcn  Expr=u(3)/sqrt(1-u(1)*u(1))
  Fcn3 : Fcn  Expr=u(4)/sqrt(1-u(1)*u(1))
  Vector Concatenate : Concatenate  NumInputs=4
  Out1 : Outport
  wires:
  In1/1 -> Fcn/1, Fcn3/1, Fcn2/1, Fcn1/1
  Fcn1/1 -> Vector Concatenate/1
  Fcn2/1 -> Vector Concatenate/2
  Fcn3/1 -> Vector Concatenate/3
  Fcn/1 -> Vector Concatenate/4
  Vector Concatenate/1 -> Out1/1

== system Bebop10_from_exp/Gate info/Yaw2Axang7/Subsystem ==
  note: u(2)/sqrt(1-u(1)*u(1)), u(3)/sqrt(1-u(1)*u(1)), u(4)/sqrt(1-u(1)*u(1)),
  In1 : Inport
  Fcn : Fcn  Expr=2*acos(u(1))
  Fcn1 : Fcn  Expr=u(2)/sqrt(1-u(1)*u(1))
  Fcn2 : Fcn  Expr=u(3)/sqrt(1-u(1)*u(1))
  Fcn3 : Fcn  Expr=u(4)/sqrt(1-u(1)*u(1))
  Vector Concatenate : Concatenate  NumInputs=4
  Out1 : Outport
  wires:
  In1/1 -> Fcn/1, Fcn3/1, Fcn2/1, Fcn1/1
  Fcn1/1 -> Vector Concatenate/1
  Fcn2/1 -> Vector Concatenate/2
  Fcn3/1 -> Vector Concatenate/3
  Fcn/1 -> Vector Concatenate/4
  Vector Concatenate/1 -> Out1/1

== system Bebop10_from_exp/Navigation/calc v/Create Path Frame ==
  Velocity Vector : Inport
  Invert 3x3 Matrix : aerolibutil/Invert  3x3 Matrix
  Make X Vector : Subsystem
  Make Y Vector : Subsystem
  Make Z Vector : Subsystem
  Matrix Concatenate : Concatenate  NumInputs=3  Mode=Multidimensional array  ConcatenateDimension=2
  Rotation Matrix : Outport
  wires:
  Velocity Vector/1 -> Make Z Vector/1(Velocity Vector), Make X Vector/1(Velocity Vector), Make Y Vector/1(Velocity Vector)
  Make Y Vector/1(Y Vector) -> Matrix Concatenate/2
  Make X Vector/1(X Vector) -> Matrix Concatenate/1
  Make Z Vector/1(Z Vector) -> Matrix Concatenate/3
  Matrix Concatenate/1 -> Invert 3x3 Matrix/1
  Invert 3x3 Matrix/1 -> Rotation Matrix/1

== system Bebop10_from_exp/Navigation/calc v/Exp offset ==
  note: y=s-(s-b) e^{-k(x-d)}
  distance : Inport
  Exp : Math  SaturateOnIntegerOverflow=on
  Gain : Gain  Gain=-1
  Minus : Sum  Inputs=-+
  Multiply : Product
  Multiply1 : Product
  Sum : Sum  Inputs=-+|
  Sum1 : Sum  Inputs=|-+
  b : Constant
  d : Constant  Value=2.5
  k : Constant  Value=-.8
  s : Constant  Value=.1
  max offset : Outport
  wires:
  distance/1 -> Sum/2
  d/1 -> Sum/1
  k/1 -> Gain/1
  Gain/1 -> Multiply/2
  Sum/1 -> Multiply/1
  Multiply/1 -> Exp/1
  b/1 -> Sum1/1
  Exp/1 -> Multiply1/1
  Sum1/1 -> Multiply1/2
  s/1 -> Minus/2, Sum1/2
  Multiply1/1 -> Minus/1
  Minus/1 -> max offset/1

== system Bebop10_from_exp/Navigation/calc v/If Action Subsystem ==
  Action Port : ActionPort  ActionType=then
  Constant : Constant
  1 : Outport
  wires:
  Constant/1 -> 1/1

== system Bebop10_from_exp/Navigation/calc v/If Action Subsystem1 ==
  spline : Inport
  Action Port : ActionPort  ActionType=else
  Add : Sum  Inputs=+++
  Dot Product1 : DotProduct  InputSameDT=on  OutDataTypeStr=Inherit: Inherit via internal rule
  Dot Product2 : DotProduct  InputSameDT=on  OutDataTypeStr=Inherit: Inherit via internal rule
  Dot Product3 : DotProduct  InputSameDT=on  OutDataTypeStr=Inherit: Inherit via internal rule
  Fcn : Fcn  Expr=(u/1.5)^2-0.01
  Minus : Sum  Inputs=-+
  Minus1 : Sum  Inputs=-+
  Minus2 : Sum  Inputs=-+
  Saturation : Saturate  UpperLimit=1.5  LowerLimit=-1
  Selector1 : Selector  NumberOfDimensions=2  IndexMode=Zero-based  InputPortWidth=3  IndexOptions=Index vector (dialog),Select all  Indices=0,[0 1 2]  OutputSizes=1,1
  Selector2 : Selector  NumberOfDimensions=2  IndexMode=Zero-based  InputPortWidth=3  IndexOptions=Index vector (dialog),Select all  Indices=1,[0 1 2]  OutputSizes=1,1
  Selector3 : Selector  NumberOfDimensions=2  IndexMode=Zero-based  InputPortWidth=3  IndexOptions=Index vector (dialog),Select all  Indices=2,[0 1 2]  OutputSizes=1,1
  Selector4 : Selector  NumberOfDimensions=2  IndexMode=Zero-based  InputPortWidth=3  IndexOptions=Index vector (dialog),Select all  Indices=3,[0 1 2]  OutputSizes=1,1
  Sqrt1 : Sqrt  SaturateOnIntegerOverflow=on
  Sqrt2 : Sqrt  SaturateOnIntegerOverflow=on
  Sqrt3 : Sqrt  SaturateOnIntegerOverflow=on
  red vel : Outport
  wires:
  Saturation/1 -> Fcn/1
  Fcn/1 -> red vel/1
  Selector2/1 -> Minus1/1, Minus/2  "P1"
  Selector3/1 -> Minus2/1, Minus1/2  "P2"
  Selector4/1 -> Minus2/2  "P3"
  spline/1 -> Selector2/1, Selector1/1, Selector4/1, Selector3/1  "spline para"
  Selector1/1 -> Minus/1  "P0"
  Minus/1 -> Dot Product3/1, Dot Product3/2
  Dot Product3/1 -> Sqrt3/1
  Sqrt3/1 -> Add/1
  Minus1/1 -> Dot Product1/1, Dot Product1/2
  Dot Product1/1 -> Sqrt1/1
  Minus2/1 -> Dot Product2/1, Dot Product2/2
  Dot Product2/1 -> Sqrt2/1
  Sqrt1/1 -> Add/2
  Sqrt2/1 -> Add/3
  Add/1 -> Saturation/1

== system Bebop10_from_exp/Navigation/calc v/calculate direction B'(d) ==
  note: B'(d) = 3(1-d)^2(P1-P0) + 6*(1-d)*d*(P2-P1) + 3d^2(P3-P2)
  spline : Inport
  d : Inport  Port=2
  Add3 : Sum  Inputs=+++
  Constant3 : Constant
  Gain : Gain  Gain=6
  Gain1 : Gain  Gain=3
  Gain2 : Gain  Gain=3
  Minus : Sum  Inputs=-+
  Minus1 : Sum  Inputs=-+
  Minus2 : Sum  Inputs=-+
  Multiply : Product
  Multiply1 : Product  Inputs=3
  Multiply8 : Product
  Power1 : Math  Operator=square  SaturateOnIntegerOverflow=on
  Power2 : Math  Operator=square  SaturateOnIntegerOverflow=on
  Selector1 : Selector  NumberOfDimensions=2  IndexMode=Zero-based  InputPortWidth=3  IndexOptions=Index vector (dialog),Select all  Indices=0,[0 1 2]  OutputSizes=1,1
  Selector2 : Selector  NumberOfDimensions=2  IndexMode=Zero-based  InputPortWidth=3  IndexOptions=Index vector (dialog),Select all  Indices=1,[0 1 2]  OutputSizes=1,1
  Selector3 : Selector  NumberOfDimensions=2  IndexMode=Zero-based  InputPortWidth=3  IndexOptions=Index vector (dialog),Select all  Indices=2,[0 1 2]  OutputSizes=1,1
  Selector4 : Selector  NumberOfDimensions=2  IndexMode=Zero-based  InputPortWidth=3  IndexOptions=Index vector (dialog),Select all  Indices=3,[0 1 2]  OutputSizes=1,1
  Sum1 : Sum  Inputs=|+-
  "old, quadratic" : Subsystem  Commented=on
  direction : Outport
  wires:
  Sum1/1 -> Multiply1/2, Power1/1
  Minus1/1 -> Multiply1/1
  Minus/1 -> Multiply/1
  Gain/1 -> Add3/2
  Gain1/1 -> Add3/3
  Multiply1/1 -> Gain/1
  Minus2/1 -> Multiply8/1
  Constant3/1 -> Sum1/1
  Multiply/1 -> Gain2/1
  Multiply8/1 -> Gain1/1
  Power2/1 -> Multiply8/2
  Power1/1 -> Multiply/2
  d/1 -> Sum1/2, Power2/1, Multiply1/3  "d"
  Gain2/1 -> Add3/1
  Add3/1 -> direction/1
  Selector1/1 -> Minus/1  "P0"
  Selector3/1 -> Minus2/1, Minus1/2  "P2"
  spline/1 -> Selector2/1, Selector1/1, Selector4/1, Selector3/1  "spline para"
  Selector2/1 -> Minus1/1, Minus/2  "P1"
  Selector4/1 -> Minus2/2  "P3"

== system Bebop10_from_exp/Navigation/calc v/min spd ==
  In1 : Inport
  Abs : Abs
  Add : Sum  Inputs=+-
  Constant : Constant  Value=0.01
  Constant1 : Constant  Value=0.5
  Minus : Sum  Inputs=+-
  Multiply : Product
  Saturation : Saturate  UpperLimit=0  LowerLimit=-1
  Scope : Scope  Commented=on  NumInputPorts=7
  Sign : Signum
  Sign1 : Signum
  Sum : Sum  Inputs=|++
  Out1 : Outport
  wires:
  In1/1 -> Scope/1, Add/1, Sign/1, Abs/1
  Abs/1 -> Minus/1
  Constant/1 -> Minus/2
  Minus/1 -> Scope/4, Saturation/1
  Saturation/1 -> Scope/5, Multiply/1
  Sum/1 -> Sign1/1
  Multiply/1 -> Scope/2, Add/2
  Add/1 -> Scope/3, Out1/1
  Constant1/1 -> Sum/2
  Sign1/1 -> Multiply/2
  Sign/1 -> Sum/1

== system Bebop10_from_exp/Navigation/calculate desired/If Action Subsystem ==
  In1 : Inport
  Action Port : ActionPort  ActionType=then
  Out1 : Outport
  wires:
  In1/1 -> Out1/1

== system Bebop10_from_exp/Navigation/calculate desired/If Action Subsystem1 ==
  In1 : Inport
  Action Port : ActionPort  ActionType=else
  Out1 : Outport
  wires:
  In1/1 -> Out1/1

== system Bebop10_from_exp/Navigation/calculate desired/calc pos B(d) ==
  note: B(d) = (1-d).^3*P0 + 3*(1-d).^2.*d*P1 + 3*(1-d).*d.^2*P2 + d.^3*P3;
  P0 : Inport
  P1 : Inport  Port=2
  P2 : Inport  Port=3
  P3 : Inport  Port=4
  d : Inport  Port=5
  Add3 : Sum  Inputs=++++
  Constant1 : Constant
  Constant2 : Constant  Value=3
  Constant3 : Constant  Value=3
  Gain : Gain  Gain=3
  Gain1 : Gain  Gain=3
  Multiply : Product
  Multiply1 : Product  Inputs=3
  Multiply8 : Product  Inputs=3
  Multiply9 : Product
  Power : Math  Operator=square  SaturateOnIntegerOverflow=on
  Power1 : Math  Operator=pow  SaturateOnIntegerOverflow=on
  Power2 : Math  Operator=square  SaturateOnIntegerOverflow=on
  Power3 : Math  Operator=pow  SaturateOnIntegerOverflow=on
  Sum1 : Sum  Inputs=|+-
  "old, quadratic" : Subsystem  Commented=on
  pos : Outport
  wires:
  Gain/1 -> Add3/2
  Gain1/1 -> Add3/3
  P1/1 -> Multiply1/1
  P0/1 -> Multiply/1
  P2/1 -> Multiply8/1
  P3/1 -> Multiply9/1
  Multiply/1 -> Add3/1
  Multiply1/1 -> Gain/1
  Multiply8/1 -> Gain1/1
  Multiply9/1 -> Add3/4
  Add3/1 -> pos/1
  Constant1/1 -> Sum1/1
  d/1 -> Sum1/2, Multiply1/3, Power2/1, Power3/1  "d"
  Power/1 -> Multiply1/2
  Power1/1 -> Multiply/2
  Power2/1 -> Multiply8/3
  Power3/1 -> Multiply9/2
  Constant2/1 -> Power1/2
  Constant3/1 -> Power3/2
  Sum1/1 -> Multiply8/2, Power/1, Power1/1

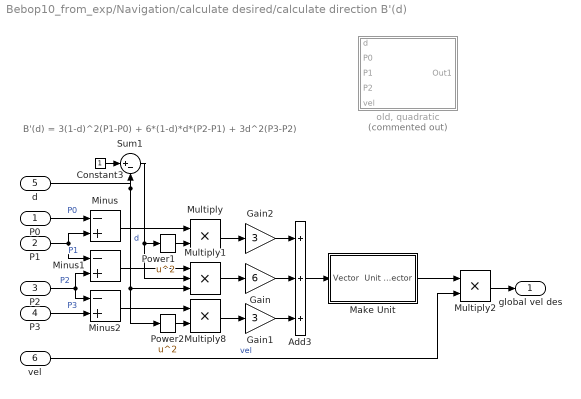
== system Bebop10_from_exp/Navigation/calculate desired/calculate direction B'(d) ==
  note: B'(d) = 3(1-d)^2(P1-P0) + 6*(1-d)*d*(P2-P1) + 3d^2(P3-P2)
  P0 : Inport
  P1 : Inport  Port=2
  P2 : Inport  Port=3
  P3 : Inport  Port=4
  d : Inport  Port=5
  vel : Inport  Port=6
  Add3 : Sum  Inputs=+++
  Constant3 : Constant
  Gain : Gain  Gain=6
  Gain1 : Gain  Gain=3
  Gain2 : Gain  Gain=3
  Make Unit : Subsystem
  Minus : Sum  Inputs=-+
  Minus1 : Sum  Inputs=-+
  Minus2 : Sum  Inputs=-+
  Multiply : Product
  Multiply1 : Product  Inputs=3
  Multiply2 : Product
  Multiply8 : Product
  Power1 : Math  Operator=square  SaturateOnIntegerOverflow=on
  Power2 : Math  Operator=square  SaturateOnIntegerOverflow=on
  Sum1 : Sum  Inputs=|+-
  "old, quadratic" : Subsystem  Commented=on
  global vel des : Outport
  wires:
  Sum1/1 -> Multiply1/2, Power1/1
  Minus1/1 -> Multiply1/1
  Minus/1 -> Multiply/1
  Gain/1 -> Add3/2
  Gain1/1 -> Add3/3
  Multiply1/1 -> Gain/1
  Minus2/1 -> Multiply8/1
  Constant3/1 -> Sum1/1
  Multiply/1 -> Gain2/1
  Multiply8/1 -> Gain1/1
  Power2/1 -> Multiply8/2
  Power1/1 -> Multiply/2
  d/1 -> Sum1/2, Power2/1, Multiply1/3  "d"
  Gain2/1 -> Add3/1
  P0/1 -> Minus/1  "P0"
  P1/1 -> Minus/2, Minus1/1  "P1"
  P2/1 -> Minus1/2, Minus2/1  "P2"
  P3/1 -> Minus2/2  "P3"
  Multiply2/1 -> global vel des/1
  Add3/1 -> Make Unit/1(Vector)
  Make Unit/1(Unit Vector) -> Multiply2/1
  vel/1 -> Multiply2/2  "vel"

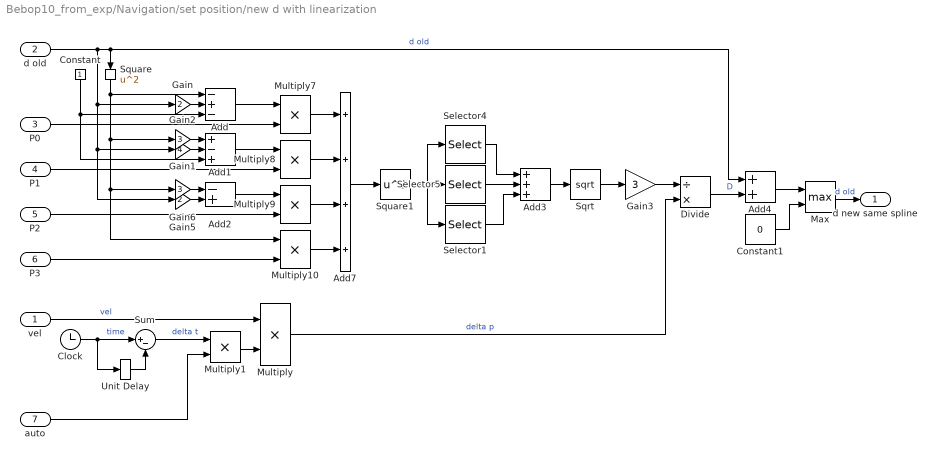
== system Bebop10_from_exp/Navigation/set position/new d with linearization ==
  vel : Inport
  d old : Inport  Port=2
  P0 : Inport  Port=3
  P1 : Inport  Port=4
  P2 : Inport  Port=5
  P3 : Inport  Port=6
  auto : Inport  Port=7
  Add : Sum  Inputs=-+-
  Add1 : Sum  Inputs=+-+
  Add2 : Sum  Inputs=-+
  Add3 : Sum  Inputs=+++
  Add4 : Sum
  Add7 : Sum  Inputs=++++
  Clock : Clock
  Constant : Constant
  Constant1 : Constant  Value=0
  Divide : Product  Inputs=/*
  Gain : Gain  Gain=2
  Gain1 : Gain  Gain=4
  Gain2 : Gain  Gain=3
  Gain3 : Gain  Gain=3
  Gain5 : Gain  Gain=2
  Gain6 : Gain  Gain=3
  Max : MinMax  Function=max  Inputs=2
  Multiply{,1,7..10} (6 alike) : Product
  Selector1 : Selector  IndexMode=Zero-based  InputPortWidth=3  IndexOptions=Index vector (dialog)  Indices=2  OutputSizes=1
  Selector4 : Selector  IndexMode=Zero-based  InputPortWidth=3  IndexOptions=Index vector (dialog)  Indices=0  OutputSizes=1
  Selector5 : Selector  IndexMode=Zero-based  InputPortWidth=3  IndexOptions=Index vector (dialog)  Indices=1  OutputSizes=1
  Sqrt : Sqrt  SaturateOnIntegerOverflow=on
  Square : Math  Operator=square  SaturateOnIntegerOverflow=on
  Square1 : Math  Operator=square  SaturateOnIntegerOverflow=on
  Sum : Sum  Inputs=|+-
  Unit Delay : UnitDelay  SampleTime=-1
  d new same spline : Outport
  wires:
  Add7/1 -> Square1/1
  Multiply8/1 -> Add7/2
  Multiply9/1 -> Add7/3
  Square/1 -> Multiply10/1, Gain6/1, Gain2/1, Add/1
  Gain/1 -> Add/2
  Constant/1 -> Add1/3, Add/3
  Gain2/1 -> Add1/1
  Gain1/1 -> Add1/2
  Gain6/1 -> Add2/1
  Gain5/1 -> Add2/2
  Multiply10/1 -> Add7/4
  Add2/1 -> Multiply9/1
  Add1/1 -> Multiply8/1
  Add/1 -> Multiply7/1
  Multiply7/1 -> Add7/1
  Selector5/1 -> Add3/2
  Gain3/1 -> Divide/1
  Divide/1 -> Add4/2  "D"
  Selector4/1 -> Add3/1
  Add3/1 -> Sqrt/1
  Square1/1 -> Selector1/1, Selector4/1, Selector5/1
  Sqrt/1 -> Gain3/1
  Selector1/1 -> Add3/3
  Add4/1 -> Max/1
  Constant1/1 -> Max/2
  P1/1 -> Multiply8/2
  P2/1 -> Multiply9/2
  P0/1 -> Multiply7/2
  Max/1 -> d new same spline/1  "d old"
  P3/1 -> Multiply10/2
  d old/1 -> Add4/1, Square/1, Gain/1, Gain5/1, Gain1/1  "d old"
  Multiply1/1 -> Multiply/2
  auto/1 -> Multiply1/2
  Clock/1 -> Unit Delay/1, Sum/1  "time"
  Multiply/1 -> Divide/2  "delta p"
  Unit Delay/1 -> Sum/2
  Sum/1 -> Multiply1/1  "delta t"
  vel/1 -> Multiply/1  "vel"

== system Bebop10_from_exp/Control/Create Path Frame/Make X Vector/Make Unit ==
  Vector : Inport
  Multiply : Product
  Reciprocal Sqrt : Sqrt  Operator=rSqrt  SaturateOnIntegerOverflow=on
  Square : Math  Operator=square  SaturateOnIntegerOverflow=on
  Sum of Elements : Sum  Inputs=+
  Unit Vector : Outport
  wires:
  Reciprocal Sqrt/1 -> Multiply/1
  Vector/1 -> Square/1, Multiply/2
  Square/1 -> Sum of Elements/1
  Multiply/1 -> Unit Vector/1
  Sum of Elements/1 -> Reciprocal Sqrt/1

== system Bebop10_from_exp/Control/Create Path Frame/Make Y Vector/Make Unit ==
  Vector : Inport
  Multiply : Product
  Reciprocal Sqrt : Sqrt  Operator=rSqrt  SaturateOnIntegerOverflow=on
  Square : Math  Operator=square  SaturateOnIntegerOverflow=on
  Sum of Elements : Sum  Inputs=+
  Unit Vector : Outport
  wires:
  Reciprocal Sqrt/1 -> Multiply/1
  Vector/1 -> Square/1, Multiply/2
  Square/1 -> Sum of Elements/1
  Multiply/1 -> Unit Vector/1
  Sum of Elements/1 -> Reciprocal Sqrt/1
